simulink model "wtd_twelve_bus_ver1"  (R2014b)
settings: Solver=ode3  StartTime=0.0  StopTime=30  FixedStep=0.002  RelTol=1e-3
undefined symbols (not defined in the file): baseSystemPower, complexPower, internalGenVoltage, j, nodeVoltage, systemFrequency, windSpeedVec, windturbKbParam
libraries: wtd_library_ver1 x16
Description:
  | Twelve Bus System
  | This model simulates nine bus system extended with DFIG (see Ref. 3 of
  | the Library  Tutorial).
  | Resulting system has 12 buses, 2 steam units, 1 hydro unit and DFIG.
  | After 3 seconds from the start of the simulation power disturbance of 10 MW is
  | introduced in the node 8.
settings Model: Creator=Jakub  LastModifiedBy=Jakub
settings DataIOCC: SignalLoggingSaveFormat=ModelDataLogs
settings OptimizationCC: ExpressionDepthLimit=2147483647
settings DebuggingCC: UnderspecifiedInitializationDetection=Classic  MergeDetectMultiDrivingBlocksExec=none  FcnCallInpInsideContextMsg=UseLocalSettings  StateNameClashWarn=warning
settings GRTTargetCC: CombineOutputUpdateFcns=off  GRTInterface=on

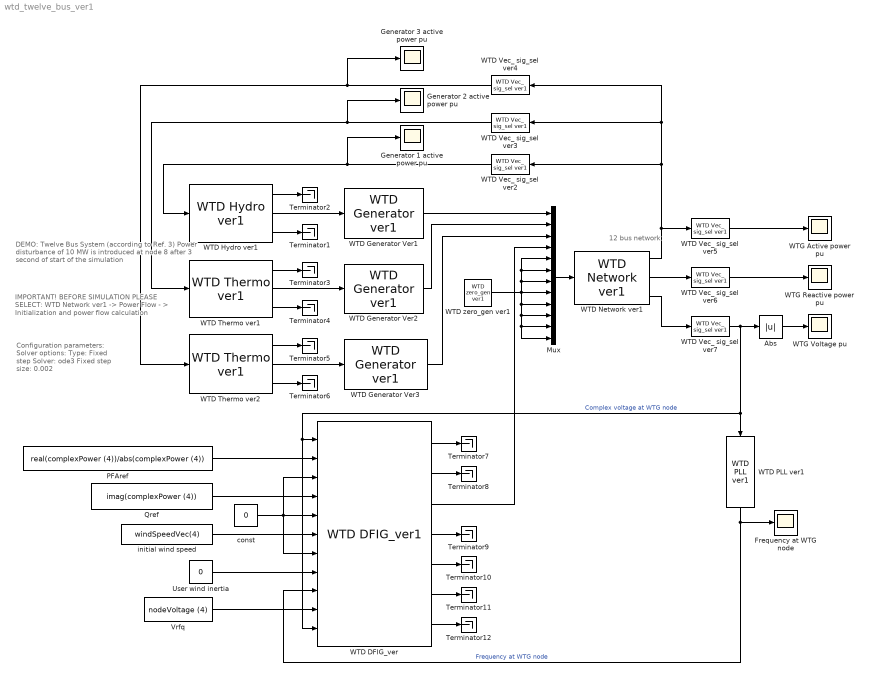
== system wtd_twelve_bus_ver1 ==
  note: DEMO: Twelve Bus System
      | (according to Ref. 3)
      | Power disturbance of 10 MW is introduced at node 8
      | after 3 second of start of the simulation
  note: IMPORTANT!
      | BEFORE SIMULATION PLEASE SELECT:
      | WTD Network ver1 -> Power Flow - >
      | Initialization and power flow calculation
  note: Configuration parameters:
      | Solver options:
      | Type: Fixed step
      | Solver: ode3
      | Fixed step size: 0.002
  note: 12 bus network
  Abs : Abs
  Frequency at WTG node : Scope
      settings: YMin=0.997  YMax=1.001  MaxDataPoints=50000
  Generator 1 active power pu : Scope
      settings: YMin=0.71  YMax=0.83  SaveName=ScopeData4  MaxDataPoints=50000
  Generator 2 active power pu : Scope
      settings: YMin=1.02  YMax=1.12  SaveName=ScopeData3  MaxDataPoints=50000
  Generator 3 active power pu : Scope
      settings: YMin=0.84  YMax=0.9  MaxDataPoints=50000
  Mux : Mux  Inputs=12
  PFAref : Constant  Value=real(complexPower (4))/abs(complexPower (4))
  Qref : Constant  Value=imag(complexPower (4))
  Terminator{1..12} (12 alike) : Terminator
  User wind inertia : Constant  Value=0
  Vrfq : Constant  Value=nodeVoltage (4)
  WTD DFIG_ver : wtd_library_ver1/WTD DFIG_ver1  co_node=4  Sbasesys=baseSystemPower  Sbasem4=100.5  wbase=2*pi*systemFrequency  H=4.94  Xsecsys=genTranReactance  Ka=windturbKaParam  Kb=windturbKbParam  Vwinit=nodeVoltage  Pelec4abs=real(complexPower)*baseSystemPower  Qgen4abs=imag(complexPower)*baseSystemPower  theta=pitchAngleVec  w=turbSpeedVec  pfaflg=0  varflg=1  apcflg=0  Kqd=0  Kpv=18  Kiv=5  Qmax=0.436  Qmin=-0.436  KVi=40  insupp=0  wi_user_GE=0  Kwi=10  Kptrq=3  Kitrq=0.6  Tpc=0.05  dbwi=0.0025  TIpwi=1  Twowi=5.5  urlwi=0.1  drlwi=-1  Pmxwi=0.1  Pmnwi=0
  WTD Generator Ver1 : wtd_library_ver1/WTD Generator ver1  co_node=1  E=internalGenVoltage  jxd=genTranReactance
  WTD Generator Ver2 : wtd_library_ver1/WTD Generator ver1  co_node=2  E=internalGenVoltage  jxd=genTranReactance
  WTD Generator Ver3 : wtd_library_ver1/WTD Generator ver1  co_node=3  E=internalGenVoltage  jxd=genTranReactance
  WTD Hydro ver1 : wtd_library_ver1/WTD Hydro ver1  co_node=1  Sbasesys=baseSystemPower  Sbasem1=247.5  wbase=2*pi*systemFrequency  H1=2364/247.5  D1=2  Pm_init_vec=real(complexPower)*baseSystemPower  delta_init_vec=angle(internalGenVoltage)  R11=0.05  r1=0.4  Tr1=8  Tf1=0.05  Tg1=0.2  VELM1=0.2  Gmax1=1  Gmin1=0  Tw1=1.2  Dturb1=0  At1=1  qNL1=0.068
  WTD Network ver1 : wtd_library_ver1/WTD Network ver1  Sbasesys=100  fsystem=50  Ydf=WTD_Y12  no_gen_co=3  no_gen_wi=1  nodes_co=[2,1,3]  xd_co=[0.1198,0.0608,0.1813]  nodes_wi=4  Pbasemw=100.5  xd_wi=0.8  Ka=0.00159  Kb=56.6  nodes_lo=[6,5,8]  Sloadabs=[90+j*30,125+j*50,100+j*35]  flttype=Power  Tfault=3  nodeadd=8  Saddabs=10  fltimp=10.32  linenumber=1  Tclear=inf  Y2df=WTD_Y12_2  absV_co=[1.025,1.04,1.025]  Sgenabs_co=[103,0,85]  wi_choice=Active_power  absV_wi=1.031  Sgenabs_wi=60  vw_vector=14  pfcalc=off  pffault=on
  WTD PLL ver1 : wtd_library_ver1/WTD PLL ver1  me_node=4  KpPLL=30  KiPLL=0  delta_init_vec=angle(nodeVoltage )  wbase=2*pi*systemFrequency
  WTD Thermo ver1 : wtd_library_ver1/WTD Thermo ver1  co_node=2  Sbasesys=baseSystemPower  Sbasem2=192  wbase=2*pi*systemFrequency  H2=640/192  D2=2  Pm_init_vec=real(complexPower)*baseSystemPower  delta_init_vec=angle(internalGenVoltage)  R2=0.05  Dt2=0  T12=0.2  T22=0.3*7  T32=7  Vmax2=1  Vmin2=0
  WTD Thermo ver2 : wtd_library_ver1/WTD Thermo ver1  co_node=3  Sbasesys=baseSystemPower  Sbasem2=128  wbase=2*pi*systemFrequency  H2=301/128  D2=2  Pm_init_vec=real(complexPower)*baseSystemPower  delta_init_vec=angle(internalGenVoltage)  R2=0.05  Dt2=0  T12=0.2  T22=0.3*7  T32=7  Vmax2=1  Vmin2=0
  WTD Vec_ sig_sel ver2 : wtd_library_ver1/WTD Vec_ sig_sel ver1  node=1
  WTD Vec_ sig_sel ver3 : wtd_library_ver1/WTD Vec_ sig_sel ver1  node=2
  WTD Vec_ sig_sel ver4 : wtd_library_ver1/WTD Vec_ sig_sel ver1  node=3
  WTD Vec_ sig_sel ver5 : wtd_library_ver1/WTD Vec_ sig_sel ver1  node=4
  WTD Vec_ sig_sel ver6 : wtd_library_ver1/WTD Vec_ sig_sel ver1  node=4
  WTD Vec_ sig_sel ver7 : wtd_library_ver1/WTD Vec_ sig_sel ver1  node=4
  WTD zero_gen ver1 : wtd_library_ver1/WTD zero_gen ver1
  WTG Active power pu : Scope
      settings: TimeRange=30  YMin=0.5775  YMax=0.6175  SaveName=ScopeData5  MaxDataPoints=50000
  WTG Reactive power pu : Scope
      settings: YMin=-0.032  YMax=-0.02  SaveName=ScopeData6  MaxDataPoints=50000
  WTG Voltage pu : Scope
      settings: YMin=1.029  YMax=1.0315  SaveName=ScopeData7  MaxDataPoints=50000
  const : Constant  Value=0
  initial wind speed : Constant  Value=windSpeedVec(4)
  wires:
  WTD Thermo ver1/2 -> WTD Generator Ver2/1
  WTD Hydro ver1/2 -> WTD Generator Ver1/1
  WTD Thermo ver2/2 -> WTD Generator Ver3/1
  WTD Hydro ver1/1 -> Terminator2/1
  WTD Hydro ver1/3 -> Terminator1/1
  WTD Thermo ver1/1 -> Terminator3/1
  WTD Thermo ver1/3 -> Terminator4/1
  WTD Thermo ver2/1 -> Terminator5/1
  WTD Thermo ver2/3 -> Terminator6/1
  Mux/1 -> WTD Network ver1/1
  WTD Generator Ver1/1 -> Mux/1
  WTD Generator Ver2/1 -> Mux/2
  WTD Generator Ver3/1 -> Mux/3
  WTD zero_gen ver1/1 -> Mux/8, Mux/6, Mux/5, Mux/7, Mux/9, Mux/10, Mux/12, Mux/11
  WTD Network ver1/1 -> WTD Vec_ sig_sel ver5/1, WTD Vec_ sig_sel ver2/1, WTD Vec_ sig_sel ver3/1, WTD Vec_ sig_sel ver4/1
  WTD Vec_ sig_sel ver2/1 -> WTD Hydro ver1/1, Generator 1 active power pu/1
  WTD Vec_ sig_sel ver3/1 -> WTD Thermo ver1/1, Generator 2 active power pu/1
  WTD Vec_ sig_sel ver4/1 -> WTD Thermo ver2/1, Generator 3 active power pu/1
  WTD Vec_ sig_sel ver5/1 -> WTG Active power pu/1
  WTD Network ver1/2 -> WTD Vec_ sig_sel ver6/1
  WTD Vec_ sig_sel ver6/1 -> WTG Reactive power pu/1
  WTD Network ver1/3 -> WTD Vec_ sig_sel ver7/1
  WTD Vec_ sig_sel ver7/1 -> Abs/1, WTD DFIG_ver/1, WTD DFIG_ver/11, WTD PLL ver1/1  "Complex voltage at WTG node"
  PFAref/1 -> WTD DFIG_ver/2
  Qref/1 -> WTD DFIG_ver/4
  initial wind speed/1 -> WTD DFIG_ver/6
  User wind inertia/1 -> WTD DFIG_ver/8
  Vrfq/1 -> WTD DFIG_ver/10
  Abs/1 -> WTG Voltage pu/1
  WTD DFIG_ver/3 -> Mux/4
  WTD DFIG_ver/1 -> Terminator7/1
  WTD PLL ver1/1 -> WTD DFIG_ver/9, Frequency at WTG node/1  "Frequency at WTG node"
  WTD DFIG_ver/2 -> Terminator8/1
  WTD DFIG_ver/4 -> Terminator9/1
  WTD DFIG_ver/5 -> Terminator10/1
  WTD DFIG_ver/6 -> Terminator11/1
  WTD DFIG_ver/7 -> Terminator12/1
  const/1 -> WTD DFIG_ver/5, WTD DFIG_ver/7, WTD DFIG_ver/3
